simulink subsystem "Navigation_Equation"  (R2022a)
settings: Solver=VariableStepAuto  StartTime=0.0  StopTime=10.0  RelTol=1e-3
undefined symbols (not defined in the file): R_earth
settings Model: Creator=Andrew Radulovich  LastModifiedBy=Andrew Radulovich

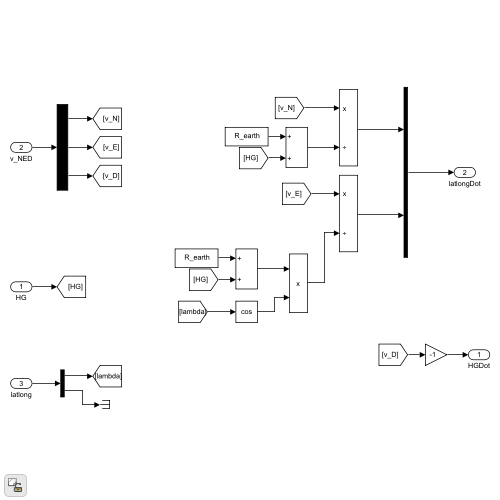
[thumbnail: Simulink's stored preview of the top-level diagram]
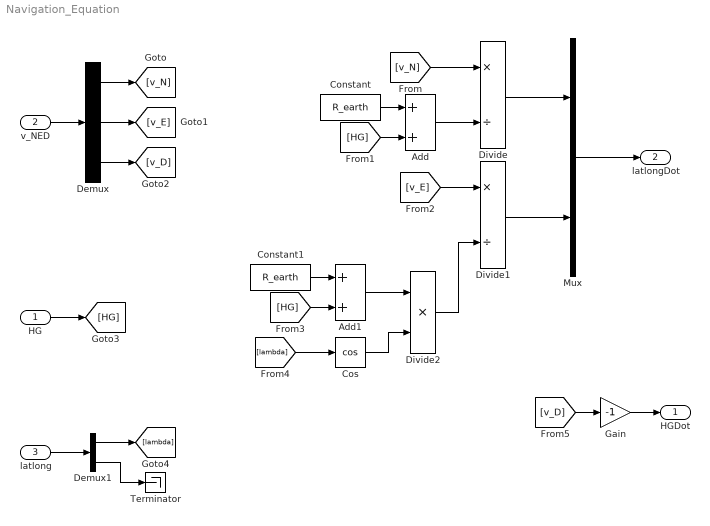
== system Navigation_Equation ==
  HG : Inport
  v_NED : Inport  Port=2
  latlong : Inport  Port=3
  Add : Sum
  Add1 : Sum
  Constant : Constant  Value=R_earth
  Constant1 : Constant  Value=R_earth
  Cos : Trigonometry  Operator=cos
  Demux : Demux  Outputs=3
  Demux1 : Demux  Outputs=2
  Divide : Product  Inputs=*/
  Divide1 : Product  Inputs=*/
  Divide2 : Product  Inputs=**
  Gain : Gain  Gain=-1
  Mux : Mux  Inputs=2
  Terminator : Terminator
  HGDot : Outport
  latlongDot : Outport  Port=2
  wires:
  v_NED/1 -> Demux/1
  Demux/1 -> [v_N]
  Demux/2 -> [v_E]
  Demux/3 -> [v_D]
  Mux/1 -> latlongDot/1
  Divide/1 -> Mux/1
  [v_N] -> Divide/1
  Add/1 -> Divide/2
  Constant/1 -> Add/1
  HG/1 -> [HG]
  [HG] -> Add/2
  Divide1/1 -> Mux/2
  [v_E] -> Divide1/1
  Add1/1 -> Divide2/1
  Divide2/1 -> Divide1/2
  Constant1/1 -> Add1/1
  [HG] -> Add1/2
  latlong/1 -> Demux1/1
  Demux1/1 -> [lambda]
  [lambda] -> Cos/1
  Cos/1 -> Divide2/2
  Demux1/2 -> Terminator/1
  [v_D] -> Gain/1
  Gain/1 -> HGDot/1
